simulink model "soc_calc"  (Simulink 8.9)
settings: Solver=ode45  StartTime=0.0  StopTime=10.0  RelTol=1e-3  EnableMultiTasking=on
settings Model: SuppressorTable=22 serialization::archive 11 0 6 0 0 0 0 0  Creator=hlopez5  LastModifiedBy=judithlopez
settings DataIOCC: SignalLoggingSaveFormat=Dataset
settings DebuggingCC: UnderspecifiedInitializationDetection=Simplified  MergeDetectMultiDrivingBlocksExec=error  SolverPrmCheckMsg=warning  FcnCallInpInsideContextMsg=error
settings GRTTargetCC: CombineOutputUpdateFcns=on  GRTInterface=off

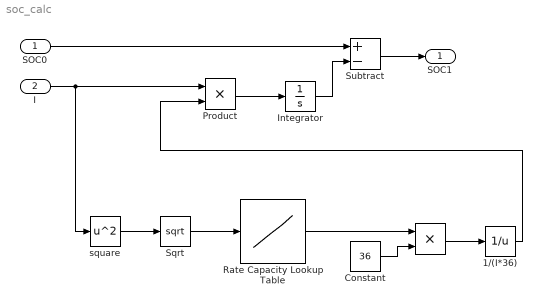
== system soc_calc ==
  SOC0 : Inport
  I : Inport  Port=2
  " " : Product
  1/(I*36) : Math  Operator=reciprocal  SaturateOnIntegerOverflow=on
  Constant : Constant  Value=36
  Integrator : Integrator
  Product : Product
  Rate Capacity Lookup Table : Lookup_n-D  NumberOfTableDimensions=1  BreakpointsForDimension1=[12.5,13,13.5]  Table=[18,9,6]  RndMeth=Simplest  InputSameDT=on
  Sqrt : Sqrt  SaturateOnIntegerOverflow=on
  Subtract : Sum  Inputs=+-
  square : Math  Operator=square  SaturateOnIntegerOverflow=on
  SOC1 : Outport
  wires:
  Subtract/1 -> SOC1/1
  SOC0/1 -> Subtract/1
  Product/1 -> Integrator/1
  Integrator/1 -> Subtract/2
  square/1 -> Sqrt/1
  Sqrt/1 -> Rate Capacity Lookup Table/1
  Rate Capacity Lookup Table/1 -> " "/1
  " "/1 -> 1/(I*36)/1
  Constant/1 -> " "/2
  1/(I*36)/1 -> Product/2
  I/1 -> Product/1, square/1
